simulink library "libUtilities"  (Simulink 8.3)
settings: Solver=ode45  StartTime=0.0  StopTime=10.0  RelTol=1e-3
undefined symbols (not defined in the file): sampPerFrame, seed
libraries: simulink x4, dspsrcs4 x3, xpclib x1
settings Model: Creator=shenoylab  LastModifiedBy=djoshea

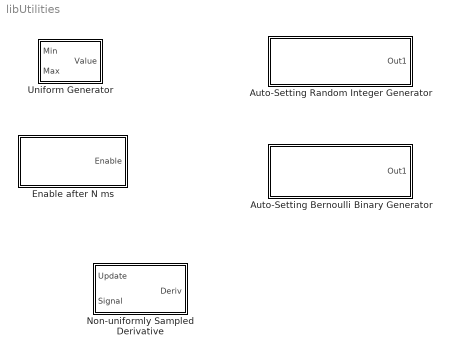
== system libUtilities ==
  Auto-Setting Bernoulli Binary Generator : Subsystem  DialogController=commDDGCreate  DialogControllerArgs=DataTag0  mask(Bernoulli Binary Generator){P=0.5, Ts=1}
      mask prompts: P "Probability of a zero:"; Ts "Sample time:"
      mask help:
      | Generate a Bernoulli random binary number.
      | To generate a vector output, specify the probability as a vector.
      mask Help: eval('blocksethelp')
      mask Display:
      | plot(0,0,100,100,[95 5 10 10 10 reshape(([85*[0:1/15:1-1/15]+10; 85*[1/15:1/15:1]+10]),1,30)],[75 75 75 70 95 90 90 90 90 80 80 80 80 90 90 80 80 80 80 90 90 90 90 80 80 80 80 90 90 90 90 80 80 90 90]);
      | disp('\nAuto-Seeding\nBernoulli Binary')
  Auto-Setting Random Integer Generator : Subsystem  mask(Random Integer Generator){mul=2^32, Ts=0.001, outDataType=uint32}
      mask prompts: mul "M-ary number:"; Ts "Sample time:"; outDataType "Output data type:"
      mask help: Generate random uniformly distributed integers in the range [0, M-1], where M is the M-ary number.
      mask Help: eval('blocksethelp')
      mask TypeOptions outDataType: double | single | int8 | uint8 | int16 | uint16 | int32 | uint32 | boolean
      mask Display:
      | plot(0,0,100,100,[95 5 10 10 10 reshape(([85*[0:1/15:1-1/15]+10; 85*[1/15:1/15:1]+10]),1,30)],[75 75 75 70 95 94 94 78 78 91 91 86 86 88 88 77 77 79 79 78 78 79 79 87 87 85 85 76 76 80 80 95 95 89 89]);
      | disp('\nAuto-Seeding\nRandom Integer')
  Enable after N ms : Subsystem  mask{const=100}
      mask prompts: const "Initial Wait Ticks"
      mask TypeOptions const:
      | Compare
      | To Constant/const
  Non-uniformly Sampled Derivative : Subsystem
  Uniform Generator : Subsystem  mask{Ts=0.001}
      mask prompts: Ts "Sample Time"
      mask help: This block auto-seeds its own uniform random number generator with a random seed at initialization.
      mask init:
      | set_param([gcb '/Generator'], 'Seed', num2str(randi(intmax)));

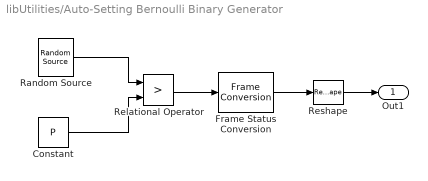
== system libUtilities/Auto-Setting Bernoulli Binary Generator ==
  Constant : Constant  Value=P  OutDataTypeStr=double  SampleTime=Ts  FramePeriod=TsMod
  Frame Status Conversion : FrameConversion  OutFrame=Sample-based
  Random Source : dspsrcs4/Random Source  SrcType=Uniform  NormMethod=Ziggurat  CltLength=12  MinVal=0  MaxVal=1  MeanVal=0  VarVal=1  RepMode=Not repeatable  rawSeed=seed  IsInherit=off  SampMode=Discrete  SampTime=Ts  SampFrame=1  DataType=Double  OutComplex=Real
  Relational Operator : RelationalOperator  Operator=>  OutDataTypeStr=float('double')  InputSameDT=on
  Reshape : Reshape  OutputDimensions=[sampPerFrame,max(length(P),length(seed))]
  Out1 : Outport
  wires:
  Random Source/1 -> Relational Operator/1
  Constant/1 -> Relational Operator/2
  Relational Operator/1 -> Frame Status Conversion/1
  Reshape/1 -> Out1/1
  Frame Status Conversion/1 -> Reshape/1

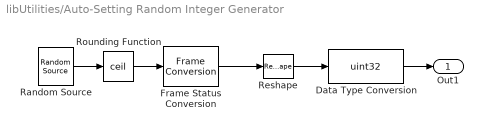
== system libUtilities/Auto-Setting Random Integer Generator ==
  Data Type Conversion : DataTypeConversion  OutDataTypeStr=uint32
  Frame Status Conversion : FrameConversion  OutFrame=Sample-based
  Random Source : dspsrcs4/Random Source  SrcType=Uniform  NormMethod=Ziggurat  CltLength=12  MinVal=-1+eps  MaxVal=mul-1  MeanVal=0  VarVal=1  RepMode=Not repeatable  rawSeed=seed  IsInherit=off  SampMode=Discrete  SampTime=Ts  SampFrame=1  DataType=Double  OutComplex=Real
  Reshape : Reshape  OutputDimensions=[sampPerFrame,max([length(mul), length(seed)])]
  Rounding Function : Rounding  Operator=ceil
  Out1 : Outport
  wires:
  Rounding Function/1 -> Frame Status Conversion/1
  Random Source/1 -> Rounding Function/1
  Frame Status Conversion/1 -> Reshape/1
  Reshape/1 -> Data Type Conversion/1
  Data Type Conversion/1 -> Out1/1

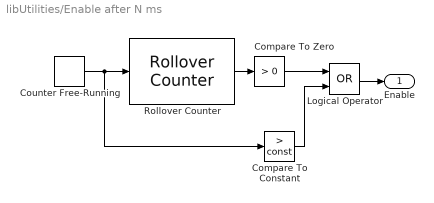
== system libUtilities/Enable after N ms ==
  Compare To Constant : simulink/Logic and Bit Operations/Compare To Constant  relop=>  const=const  OutDataTypeStr=uint8
  Compare To Zero : simulink/Logic and Bit Operations/Compare To Zero  relop=>  OutDataTypeStr=uint8
  Counter Free-Running : simulink/Sources/Counter Free-Running  NumBits=16  tsamp=-1
  Logical Operator : Logic  Operator=OR  AllPortsSameDT=off  OutDataTypeStr=boolean
  Rollover Counter : xpclib/Incremental Encoder/Utilities/Rollover/Rollover Counter  InitialValue=0  RolloverThreshold=2^15
  Enable : Outport
  wires:
  Logical Operator/1 -> Enable/1
  Compare To Constant/1 -> Logical Operator/2
  Compare To Zero/1 -> Logical Operator/1
  Rollover Counter/1 -> Compare To Zero/1
  Counter Free-Running/1 -> Compare To Constant/1, Rollover Counter/1

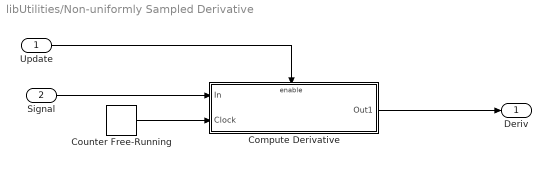
== system libUtilities/Non-uniformly Sampled Derivative ==
  Update : Inport
  Signal : Inport  Port=2
  Compute Derivative : Subsystem
  Counter Free-Running : simulink/Sources/Counter Free-Running  NumBits=32  tsamp=-1
  Deriv : Outport
  wires:
  Counter Free-Running/1 -> Compute Derivative/2(Clock)
  Compute Derivative/1(Out1) -> Deriv/1
  Signal/1 -> Compute Derivative/1(In)
  Update/1 -> Compute Derivative/Enable

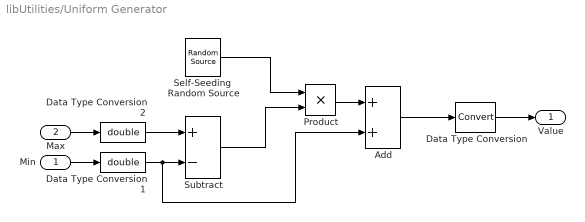
== system libUtilities/Uniform Generator ==
  Min : Inport
  Max : Inport  Port=2
  Add : Sum
  Data Type Conversion : DataTypeConversion
  Data Type Conversion1 : DataTypeConversion  OutDataTypeStr=double
  Data Type Conversion2 : DataTypeConversion  OutDataTypeStr=double
  Product : Product  RndMeth=Zero
  Self-Seeding  Random Source : dspsrcs4/Random Source  SrcType=Uniform  NormMethod=Ziggurat  CltLength=12  MinVal=0  MaxVal=1  MeanVal=0  VarVal=1  RepMode=Not repeatable  rawSeed=1  IsInherit=off  SampMode=Discrete  SampTime=Ts  SampFrame=1  DataType=Double  OutComplex=Real
  Subtract : Sum  Inputs=+-
  Value : Outport
  wires:
  Max/1 -> Data Type Conversion2/1
  Add/1 -> Data Type Conversion/1
  Self-Seeding  Random Source/1 -> Product/1
  Min/1 -> Data Type Conversion1/1
  Subtract/1 -> Product/2
  Product/1 -> Add/1
  Data Type Conversion/1 -> Value/1
  Data Type Conversion1/1 -> Subtract/2, Add/2
  Data Type Conversion2/1 -> Subtract/1

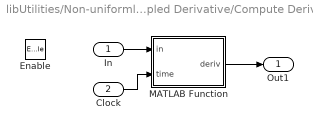
== system libUtilities/Non-uniformly Sampled Derivative/Compute Derivative ==
  In : Inport
  Clock : Inport  Port=2  OutDataTypeStr=uint32
  Enable : EnablePort
  MATLAB Function : MATLAB Function  TreatAsAtomicUnit=on
  Out1 : Outport  InitialOutput=0
  wires:
  Clock/1 -> MATLAB Function/2(time)
  MATLAB Function/1(deriv) -> Out1/1
  In/1 -> MATLAB Function/1(in)

== matlab function Non-uniformly Sampled Derivative/Compute Derivative/MATLAB Function ==
  data: in input double; deriv output double; time input double
function deriv = fcn(in, time)
%#codegen

persistent pIn;
if isempty(pIn)
    pIn = in;
end

persistent pTime;
if isempty(pTime)
    pTime = time - uint32(1);
end

if double(time - pTime) > 0
    deriv = (double(in) - double(pIn)) / double(time - pTime);
else
    deriv = 0;
end

pIn = in;
pTime = time;
